simulink model "midRangeSim"  (R2018a)
settings: Solver=VariableStepAuto  StartTime=0.0  StopTime=10.0  RelTol=1e-3
values from neighbouring files (symbols this model uses):
  GPC = gpc_tf2ss_midRange(Pz,C,delta,n,nu)    [midRange.m]
  Ke = K(nin,:)*GPC.E    [midRange.m]
  Kf = K(nin,:)*GPC.F    [midRange.m]
  Kr = K(nin,:)*w    [midRange.m]
  Ur = 0.1*ones(n,1)    [midRange.m]
libraries: cstblocks x1
settings Model: Creator=marcus  LastModifiedBy=marcus

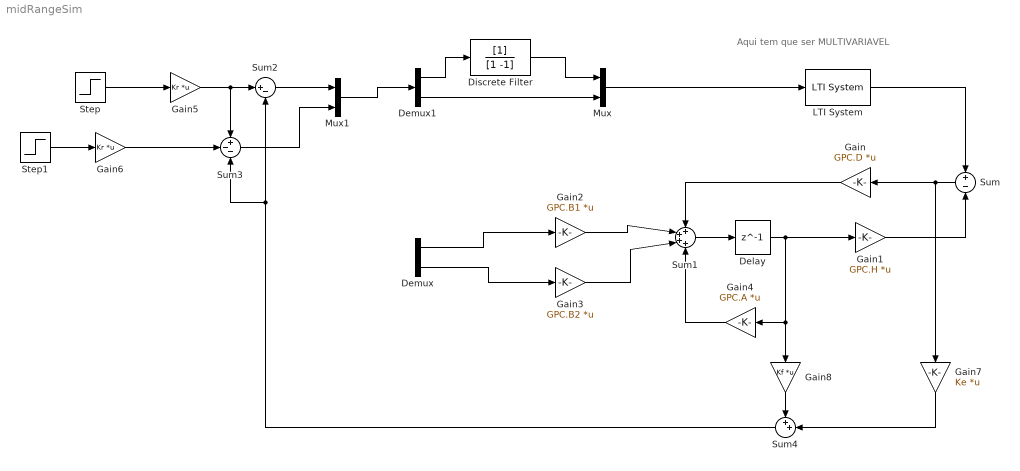
== system midRangeSim ==
  note: Aqui tem que ser MULTIVARIAVEL
  Delay : Delay  DelayLength=1
  Demux : Demux  Outputs=2
  Demux1 : Demux  Outputs=2
  Discrete Filter : DiscreteFilter  Denominator=[1 -1]
  Gain : Gain  Gain=GPC.D  Multiplication=Matrix(K*u)
  Gain1 : Gain  Gain=GPC.H  Multiplication=Matrix(K*u)
  Gain2 : Gain  Gain=GPC.B1  Multiplication=Matrix(K*u)
  Gain3 : Gain  Gain=GPC.B2  Multiplication=Matrix(K*u)
  Gain4 : Gain  Gain=GPC.A  Multiplication=Matrix(K*u)
  Gain5 : Gain  Gain=Kr  Multiplication=Matrix(K*u)
  Gain6 : Gain  Gain=Kr  Multiplication=Matrix(K*u)
  Gain7 : Gain  Gain=Ke  Multiplication=Matrix(K*u)
  Gain8 : Gain  Gain=Kf  Multiplication=Matrix(K*u)
  LTI System : cstblocks/LTI System  sys=Pn  IC=[]
  Mux : Mux  Inputs=2
  Mux1 : Mux  Inputs=2
  Step : Step  SampleTime=0
  Step1 : Step  After=Ur  SampleTime=0
  Sum : Sum  Inputs=+-
  Sum1 : Sum  Inputs=++++
  Sum2 : Sum  Inputs=|+-
  Sum3 : Sum  Inputs=+--
  Sum4 : Sum  Inputs=++|
  wires:
  Mux/1 -> LTI System/1
  LTI System/1 -> Sum/1
  Sum/1 -> Gain/1, Gain7/1
  Gain1/1 -> Sum/2
  Gain/1 -> Sum1/1
  Gain2/1 -> Sum1/2
  Gain3/1 -> Sum1/3
  Sum1/1 -> Delay/1
  Delay/1 -> Gain8/1, Gain4/1, Gain1/1
  Gain4/1 -> Sum1/4
  Demux/1 -> Gain2/1
  Demux/2 -> Gain3/1
  Gain7/1 -> Sum4/2
  Gain8/1 -> Sum4/1
  Gain5/1 -> Sum3/1, Sum2/1
  Step/1 -> Gain5/1
  Discrete Filter/1 -> Mux/1
  Demux1/1 -> Discrete Filter/1
  Demux1/2 -> Mux/2
  Sum4/1 -> Sum3/3, Sum2/2
  Gain6/1 -> Sum3/2
  Step1/1 -> Gain6/1
  Sum2/1 -> Mux1/1
  Sum3/1 -> Mux1/2
  Mux1/1 -> Demux1/1
